simulink model "simulinkM11"  (R2021b)
settings: Solver=VariableStepAuto  StartTime=0.0  StopTime=3  RelTol=1e-3
values from neighbouring files (symbols this model uses):
  K1 = wn^2    [zadanieM11.m]
  K2 = 2*zeta*wn-1    [zadanieM11.m]
  wn = BW/sqrt((1-2*zeta^2) + sqrt(4*zeta^4 - 4*zeta^2 + 2))    [zadanieM10.m]    (also in zadanieM11.m = pi/(tp * sqrt(1-zeta^2)))
  zeta = rzeta(4)    [zadanieM10.m]    (also in zadanieM11.m = sqrt(1/(a^2 + 1)))
settings Model: Creator=Studenci  LastModifiedBy=Studenci

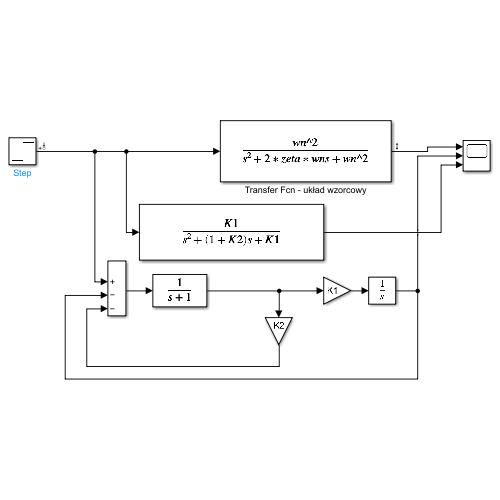
[thumbnail: Simulink's stored preview of the top-level diagram]
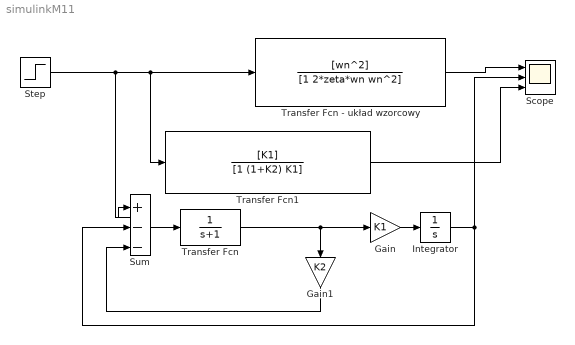
== system simulinkM11 ==
  Gain : Gain  Gain=K1
  Gain1 : Gain  Gain=K2
  Integrator : Integrator
  Scope : Scope  NumInputPorts=3
  Step : Step  SampleTime=0
  Sum : Sum  Inputs=|+--
  Transfer Fcn : TransferFcn  Denominator=[1 1]
  Transfer Fcn - układ wzorcowy : TransferFcn  Numerator=[wn^2]  Denominator=[1 2*zeta*wn wn^2]
  Transfer Fcn1 : TransferFcn  Numerator=[K1]  Denominator=[1 (1+K2) K1]
  wires:
  Step/1 -> Sum/1, Transfer Fcn1/1, Transfer Fcn - układ wzorcowy/1
  Transfer Fcn - układ wzorcowy/1 -> Scope/1
  Gain1/1 -> Sum/3
  Integrator/1 -> Scope/2, Sum/2
  Transfer Fcn1/1 -> Scope/3
  Sum/1 -> Transfer Fcn/1
  Gain/1 -> Integrator/1
  Transfer Fcn/1 -> Gain/1, Gain1/1
